simulink subsystem "Subsystem"  (R2020a)
settings: Solver=VariableStepAuto  StartTime=0.0  StopTime=10.0  RelTol=1e-3
libraries: simulink x1
settings Model: Creator=Atharv Sharma  LastModifiedBy=Atharv Sharma

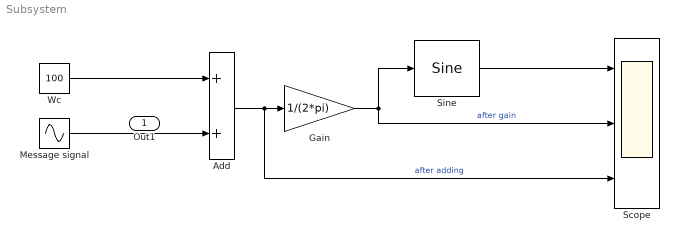
== system Subsystem ==
  Add : Sum
  Gain : Gain  Gain=1/(2*pi)
  Message signal : Sin  Amplitude=30  Frequency=10  SampleTime=.0001
  Scope : Scope  NumInputPorts=3
  Sine : simulink/Lookup Tables/Sine  Formula=sin(2*pi*u)  NumDataPoints=(2^5)+1  OutputWordLength=16  InternalRulePriority=Speed
  Wc : Constant  Value=100  SampleTime=.0001
  Out1 : Outport
  wires:
  Message signal/1 -> Add/2
  Sine/1 -> Scope/1
  Gain/1 -> Sine/1, Scope/2  "after gain"
  Add/1 -> Gain/1, Scope/3  "after adding"
  Wc/1 -> Add/1
